simulink model "fourdrive_test"  (R2022b)
settings: Solver=FixedStepDiscrete  StartTime=0.0  StopTime=10.0  FixedStep=0.001  RelTol=1e-3  EnableMultiTasking=on
PreLoadFcn:
  | PowerOn_data
InitFcn:
  | EcoCoder_PreCheckLic();
undefined symbols (not defined in the file or in its folder): HV_Botton, Inverter_Button, SC_Closed
libraries: CoderSF_BSW_Libs x113, SF_CanService_Libs x24, CoderSF_ADC2Volt_Libs x10, simulink x2
(part 1 of 2)
settings Model: Param_HCUVersion=EV22297A  Creator=hxf  LastModifiedBy=34547
settings SolverCC: AlgebraicLoopSolver=TrustRegion  AutoInsertRateTranBlk=on
settings DataIOCC: SaveFormat=Structure  SignalLoggingSaveFormat=ModelDataLogs  SaveOutput=off  SignalLogging=off  DSMLogging=off  SaveTime=off  ReturnWorkspaceOutputs=off
settings OptimizationCC: DefaultParameterBehavior=Inlined  InlineInvariantSignals=on  EnhancedBackFolding=on  StrengthReduction=on  EnableMemcpy=off  PassReuseOutputArgsAs=Individual arguments  EfficientFloat2IntCast=on  LifeSpan=1  SimCompilerOptimization=on  OptimizeBlockOrder=speed  DifferentSizesBufferReuse=on  EfficientTunableParamExpr=on
settings DebuggingCC: AlgebraicLoopMsg=none  ArtificialAlgebraicLoopMsg=none  SaveWithDisabledLinksMsg=none  SaveWithParameterizedLinksMsg=none  CheckSSInitialOutputMsg=off  UnderspecifiedInitializationDetection=Classic  SignalResolutionControl=TryResolveAll  BlockPriorityViolationMsg=error  MinStepSizeMsg=none  InheritedTsInSrcMsg=none  MultiTaskDSMMsg=none  MultiTaskCondExecSysMsg=none  MultiTaskRateTransMsg=warning  TasksWithSamePriorityMsg=none  SigSpecEnsureSampleTimeMsg=none  IntegerOverflowMsg=error  Int32ToFloatConvMsg=none  ParameterPrecisionLossMsg=none  ParameterTunabilityLossMsg=none  FixptConstOverflowMsg=error  FcnCallInpInsideContextMsg=warning  UnconnectedInputMsg=error  UnconnectedOutputMsg=error  UnconnectedLineMsg=error  FrameProcessingCompatibilityMsg=none  BusObjectLabelMismatch=none  RootOutportRequireBusObject=none  UnknownTsInhSupMsg=none  ModelReferenceDataLoggingMessage=none  OperatingPointInterfaceChecksumMismatchMsg=none  SFUnusedDataAndEventsDiag=none  SFUnexpectedBacktrackingDiag=none  SFInvalidInputDataAccessInChartInitDiag=none  SFNoUnconditionalDefaultTransitionDiag=none  SFTransitionOutsideNaturalParentDiag=none  SFUnreachableExecutionPathDiag=none  SFMachineParentedDataDiag=warning  ArithmeticOperatorsInVariantConditions=warning
settings HardwareCC: ProdBitPerPointer=32  ProdBitPerSizeT=32  ProdBitPerPtrDiffT=32  ProdLargestAtomicFloat=None  ProdWordSize=32  ProdHWDeviceType=Infineon->TriCore
settings ModelReferenceCC: UpdateModelReferenceTargets=Force  EnableRefExpFcnMdlSchedulingChecks=on  ModelReferenceNumInstancesAllowed=Single  PropagateSignalLabelsOutOfModel=off
settings SFSimCC: SFSimEcho=off  MATLABDynamicMemAlloc=off  CustomCodeUndefinedFunction=UseInterfaceOnly
settings RTWCC: Description=Ecotrons TC27x  SystemTargetFile=EcoCoderTC27x.tlc  GenerateMakefile=off  TemplateMakefile=ert_default_tmf  RTWVerbose=off  RetainRTWFile=on  RTWCompilerOptimization=on
settings CodeAppCC: IgnoreCustomStorageClasses=off  OperatorAnnotations=on  CustomSymbolStrGlobalVar=$N$M  CustomSymbolStrType=$N$M  CustomSymbolStrFcn=$N$M  CustomSymbolStrFcnArg=$N$M  CustomSymbolStrBlkIO=$N$M  CustomSymbolStrMacro=$N$M
settings STFCustomTargetCC: UtilityFuncGeneration=Shared location  MultiwordLength=256  IncludeMdlTerminateFcn=off  CombineOutputUpdateFcns=on  SuppressErrorStatus=on  ERTCustomFileBanners=on  SupportComplex=off  SupportContinuousTime=off  SupportNonInlinedSFcns=off  MATLABClassNameForMDSCustomization=Simulink.SoftwareTarget.ERTCustomization  SystemTargetFile=EcoCoderTC27x.tlc
settings ERTTargetCC: UtilityFuncGeneration=Shared location  ParMdlRefBuildCompliant=off  CompOptLevelCompliant=off  ConcurrentExecutionCompliant=off  IncludeMdlTerminateFcn=off  SuppressErrorStatus=on  SupportComplex=off  RemoveResetFunc=off  ModelStepFunctionPrototypeControlCompliant=off  CPPClassGenCompliant=off  UseToolchainInfoCompliant=off  GenerateASAP2=on  InlinedParameterPlacement=NonHierarchical  ERTCustomFileTemplate=MPC5644A_file_process.tlc  ERTFilePackagingFormat=Compact  PreserveIfCondition=on  ConvertIfToSwitch=off  PreserveExternInFcnDecls=off  SuppressUnreachableDefaultCases=off

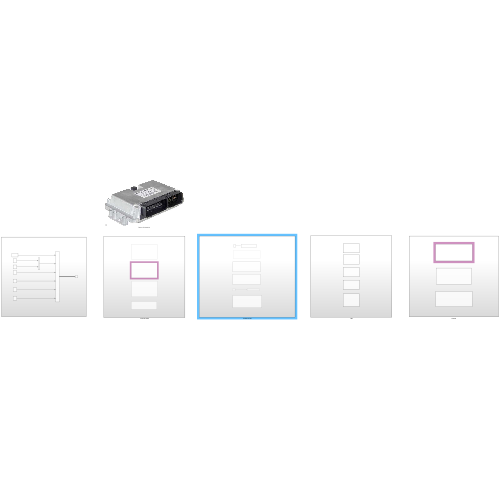
[thumbnail: Simulink's stored preview of the top-level diagram]
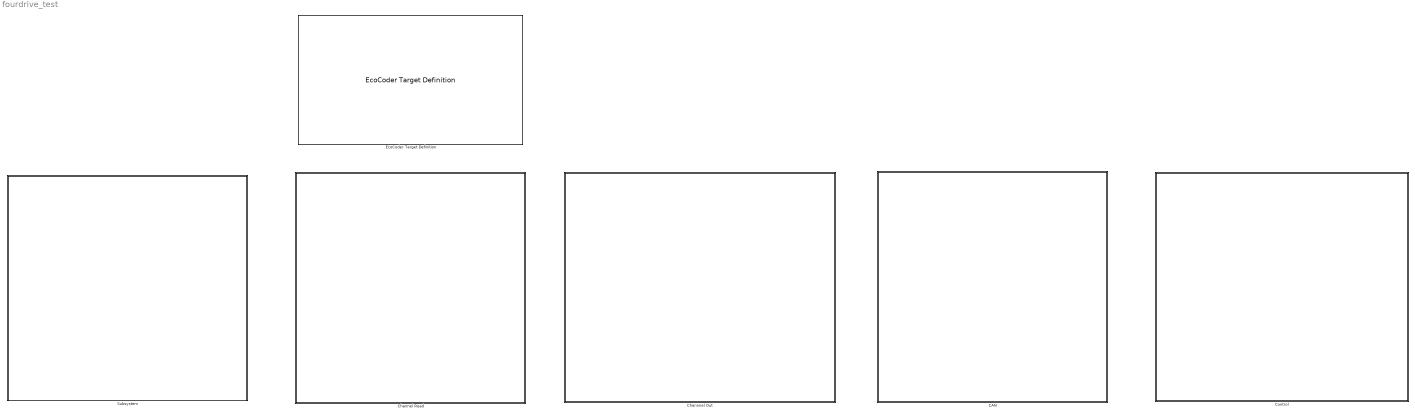
== system fourdrive_test ==
  CAN : Subsystem
  Channel Read : Subsystem
  Channnel Out : Subsystem
  Control : Subsystem
  EcoCoder Target Definition : CoderSF_BSW_Libs/EcoCoder Target Definition  targetECU=EV22297A  EcoCoderBlockID=T001_Target  enNoTriggerCall=on  flgBlockReduction=on  flgShowDebugDisp=off  flgDisTargetOutFIleCounter=off  flgClearAllOldFiles=on  tc275_cal_len=hex2dec('00008000')  ipVal='192.168.0.123'  userName='nvidia'  passWord='nvidia'  workSpace='~/cmake_ws'  libraryLink=''  enExt=on  portExt=17725  internal_flash=[hex2dec('00020000'),hex2dec('000E0000')]  cal_rom_phy=[hex2dec('00010000'),hex2dec('00002000')]  cal_ram_wp=[hex2dec('4000F000'),hex2dec('00002000')]  cal_ram_msm=[hex2dec('40000000'),hex2dec('00002000')]  var_ram_wp=[hex2dec('40002000'),hex2dec('0000D000')]  write_back_fixed_ram=[hex2dec('40011000'),hex2dec('00001000')]  write_back_unfixed_ram=[hex2dec('40012000'),hex2dec('00001000')]  stack=[hex2dec('40013000'),hex2dec('00001000')]
      settings: AttributesFormatString=Target :%<targetECU>
  Subsystem : Subsystem

== system fourdrive_test/CAN ==
  CAN Definition : Subsystem
  CAN Read : Subsystem
  CAN Write : Subsystem
  Fixed CCP Slave Definition : CoderSF_BSW_Libs/CCP/Fixed CCP Slave Definition  ccp_enSet=on  ccp_disASW=off  channel=CAN_B  stationaddressSet=hex2dec('0112')  croidSet=hex2dec('200')  dtoidSet=hex2dec('201')  daqidSet=[hex2dec('210') hex2dec('211') hex2dec('212') hex2dec('213')]  daqpidSet=[hex2dec('0') hex2dec('0') hex2dec('0') hex2dec('0')]  daqlenSet=[hex2dec('A') hex2dec('20') hex2dec('30') hex2dec('50')]  daqperSet=[10 20 100 200]  EcoCoderBlockID=C002_CCP21Conf
  Write CAN Measurement : Subsystem

== system fourdrive_test/Channel Read ==
  ADC : Subsystem
  DI : Subsystem

== system fourdrive_test/Channnel Out ==
  Constant1 : Constant  OutDataTypeStr=boolean
  DC板 : Subsystem
  Power Control Output : CoderSF_BSW_Libs/System Management Blocks/Power Control Output  channel=PWR5V3
  Terminator : Terminator
  水泵风扇 : Subsystem
  蜂鸣器 : Subsystem
  wires:
  Constant1/1 -> Power Control Output/1
  [Brake_angle_percent] -> Terminator/1

== system fourdrive_test/Control ==
  Motor_Enable : Subsystem
  StateMachine : Subsystem
  Torque_Control : Subsystem

== system fourdrive_test/Subsystem ==
  Bus Creator : BusCreator  Inputs=Wheelbase,Distribution of Axle Load,Front Length,Rear Length,Front Track Width,Rear Track Width
  Divide : Product  Inputs=*/
  Front Length : Constant  Value=0.79
  Front Mass : Constant  Value=110
  Front Track Width : Constant  Value=1.2
  Rear Length : Constant  Value=0.79
  Rear Mass : Constant  Value=135
  Rear Track Width : Constant  Value=1.16
  Terminator : Terminator
  Wheelbase : Constant  Value=1.58
  wires:
  Front Mass/1 -> Divide/1
  Rear Mass/1 -> Divide/2
  Divide/1 -> Bus Creator/2  "Distribution of Axle Load"
  Wheelbase/1 -> Bus Creator/1  "Wheelbase"
  Front Length/1 -> Bus Creator/3  "Front Length"
  Rear Length/1 -> Bus Creator/4  "Rear Length"
  Front Track Width/1 -> Bus Creator/5  "Front Track Width"
  Rear Track Width/1 -> Bus Creator/6  "Rear Track Width"
  Bus Creator/1 -> Terminator/1

== system fourdrive_test/CAN/CAN Definition ==
  CAN Channel Definition : CoderSF_BSW_Libs/CAN/CAN Channel Definition  channel=CAN_A  can_en=on  can_idfilter=off  can_rxextended=off  can_rxMask=hex2dec('7ff')  can_rxID=hex2dec('100')  can_baudrateIndex=250  can_txbuffer_size=200  can_rxbuffer_size=1  can_en_fd=off  nominalSamplePoint=7500  can_baudrateIndex_data=500  fastSamplePoint=7500  canfd_txbuffer_size=5  EcoCoderBlockID=C001_CANDef
  CAN Channel Definition1 : CoderSF_BSW_Libs/CAN/CAN Channel Definition  channel=CAN_B  can_en=on  can_idfilter=off  can_rxextended=off  can_rxMask=hex2dec('7ff')  can_rxID=hex2dec('100')  can_baudrateIndex=500  can_txbuffer_size=200  can_rxbuffer_size=1  can_en_fd=off  nominalSamplePoint=7500  can_baudrateIndex_data=500  fastSamplePoint=7500  canfd_txbuffer_size=5  EcoCoderBlockID=C001_CANDef
  CAN Channel Definition2 : CoderSF_BSW_Libs/CAN/CAN Channel Definition  channel=CAN_C  can_en=on  can_idfilter=off  can_rxextended=off  can_rxMask=hex2dec('7ff')  can_rxID=hex2dec('100')  can_baudrateIndex=500  can_txbuffer_size=20  can_rxbuffer_size=1  can_en_fd=off  nominalSamplePoint=7500  can_baudrateIndex_data=500  fastSamplePoint=7500  canfd_txbuffer_size=5  EcoCoderBlockID=C001_CANDef
  CAN Channel Definition3 : CoderSF_BSW_Libs/CAN/CAN Channel Definition  channel=CAN_D  can_en=on  can_idfilter=off  can_rxextended=off  can_rxMask=hex2dec('7ff')  can_rxID=hex2dec('100')  can_baudrateIndex=500  can_txbuffer_size=20  can_rxbuffer_size=1  can_en_fd=off  nominalSamplePoint=7500  can_baudrateIndex_data=500  fastSamplePoint=7500  canfd_txbuffer_size=5  EcoCoderBlockID=C001_CANDef
  CAN Channel Definition4 : CoderSF_BSW_Libs/CAN/CAN Channel Definition  channel=CAN_E  can_en=on  can_idfilter=off  can_rxextended=off  can_rxMask=hex2dec('7ff')  can_rxID=hex2dec('100')  can_baudrateIndex=250  can_txbuffer_size=20  can_rxbuffer_size=1  can_en_fd=off  nominalSamplePoint=7500  can_baudrateIndex_data=500  fastSamplePoint=7500  canfd_txbuffer_size=5  EcoCoderBlockID=C001_CANDef

== system fourdrive_test/CAN/CAN Read ==
  BMS_CAN : Subsystem
  Motor_CAN : Subsystem

== system fourdrive_test/CAN/CAN Write ==
  Send_To_Inverter : Subsystem
  Send_To_Recorder : Subsystem

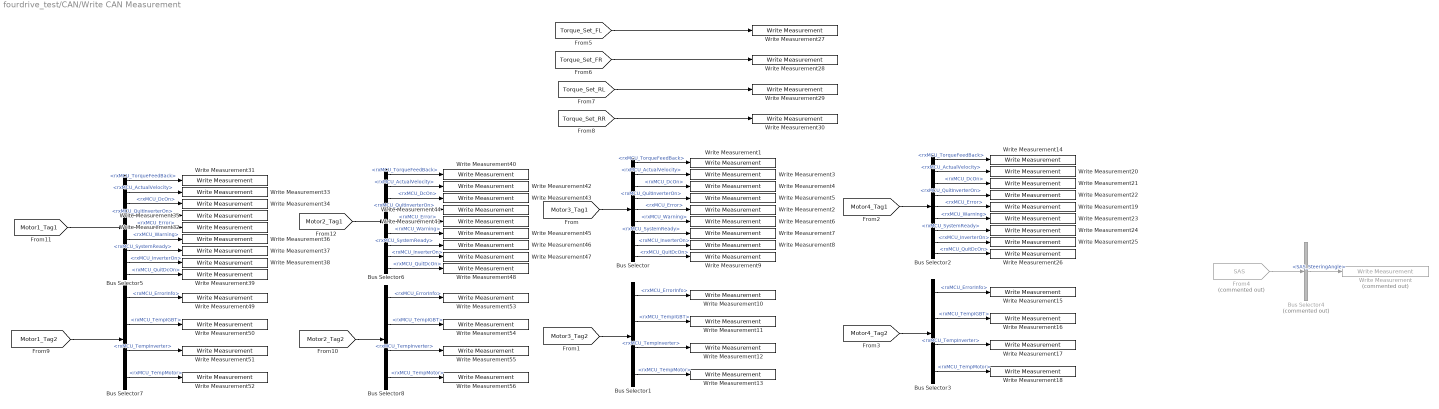
== system fourdrive_test/CAN/Write CAN Measurement ==
  Bus Selector{,2,5..6} (4 alike) : BusSelector  OutputSignals=rxMCU_TorqueFeedBack,rxMCU_ActualVelocity,rxMCU_DcOn,rxMCU_QuitInverterOn,rxMCU_Error,rxMCU_Warning,rxMCU_SystemReady,rxMCU_InverterOn,rxMCU_QuitDcOn
  Bus Selector{1,3,7..8} (4 alike) : BusSelector  OutputSignals=rxMCU_ErrorInfo,rxMCU_TempIGBT,rxMCU_TempInverter,rxMCU_TempMotor
  Bus Selector4 : BusSelector  Commented=on  OutputSignals=SAS_SteeringAngle
  From4 : From  Commented=on  GotoTag=SAS  TagVisibility=global
  Write Measurement : CoderSF_BSW_Libs/Calibration & Measurement/Write Measurement  Commented=on  variable_name=Steering_Angle  variable_value=0  variable_type=single  numD=1  unitStr=""  descStr=""
      settings: AttributesFormatString=type:%<variable_type> Dimensions:%<numD>
  Write Measurement1 : CoderSF_BSW_Libs/Calibration & Measurement/Write Measurement  variable_name=RL_Actual_Torque  variable_value=0  variable_type=single  numD=1  unitStr=""  descStr=""
      settings: AttributesFormatString=type:%<variable_type> Dimensions:%<numD>
  Write Measurement10 : CoderSF_BSW_Libs/Calibration & Measurement/Write Measurement  variable_name=RL_Error_Info  variable_value=0  variable_type=uint16  numD=1  unitStr=""  descStr=""
      settings: AttributesFormatString=type:%<variable_type> Dimensions:%<numD>
  Write Measurement11 : CoderSF_BSW_Libs/Calibration & Measurement/Write Measurement  variable_name=RL_TempIGBT  variable_value=0  variable_type=single  numD=1  unitStr=""  descStr=""
      settings: AttributesFormatString=type:%<variable_type> Dimensions:%<numD>
  Write Measurement12 : CoderSF_BSW_Libs/Calibration & Measurement/Write Measurement  variable_name=RL_TempInverter  variable_value=0  variable_type=single  numD=1  unitStr=""  descStr=""
      settings: AttributesFormatString=type:%<variable_type> Dimensions:%<numD>
  Write Measurement13 : CoderSF_BSW_Libs/Calibration & Measurement/Write Measurement  variable_name=RL_TempMotor  variable_value=0  variable_type=single  numD=1  unitStr=""  descStr=""
      settings: AttributesFormatString=type:%<variable_type> Dimensions:%<numD>
  Write Measurement14 : CoderSF_BSW_Libs/Calibration & Measurement/Write Measurement  variable_name=RR_Actual_Torque  variable_value=0  variable_type=single  numD=1  unitStr=""  descStr=""
      settings: AttributesFormatString=type:%<variable_type> Dimensions:%<numD>
  Write Measurement15 : CoderSF_BSW_Libs/Calibration & Measurement/Write Measurement  variable_name=RR_Error_Info  variable_value=0  variable_type=uint16  numD=1  unitStr=""  descStr=""
      settings: AttributesFormatString=type:%<variable_type> Dimensions:%<numD>
  Write Measurement16 : CoderSF_BSW_Libs/Calibration & Measurement/Write Measurement  variable_name=RR_TempIGBT  variable_value=0  variable_type=single  numD=1  unitStr=""  descStr=""
      settings: AttributesFormatString=type:%<variable_type> Dimensions:%<numD>
  Write Measurement17 : CoderSF_BSW_Libs/Calibration & Measurement/Write Measurement  variable_name=RR_TempInverter  variable_value=0  variable_type=single  numD=1  unitStr=""  descStr=""
      settings: AttributesFormatString=type:%<variable_type> Dimensions:%<numD>
  Write Measurement18 : CoderSF_BSW_Libs/Calibration & Measurement/Write Measurement  variable_name=RR_TempMotor  variable_value=0  variable_type=single  numD=1  unitStr=""  descStr=""
      settings: AttributesFormatString=type:%<variable_type> Dimensions:%<numD>
  Write Measurement19 : CoderSF_BSW_Libs/Calibration & Measurement/Write Measurement  variable_name=RR_Error  variable_value=0  variable_type=boolean  numD=1  unitStr=""  descStr=""
      settings: AttributesFormatString=type:%<variable_type> Dimensions:%<numD>
  Write Measurement2 : CoderSF_BSW_Libs/Calibration & Measurement/Write Measurement  variable_name=RL_Error  variable_value=0  variable_type=boolean  numD=1  unitStr=""  descStr=""
      settings: AttributesFormatString=type:%<variable_type> Dimensions:%<numD>
  Write Measurement20 : CoderSF_BSW_Libs/Calibration & Measurement/Write Measurement  variable_name=RR_Actual_Velocity  variable_value=0  variable_type=int16  numD=1  unitStr=""  descStr=""
      settings: AttributesFormatString=type:%<variable_type> Dimensions:%<numD>
  Write Measurement21 : CoderSF_BSW_Libs/Calibration & Measurement/Write Measurement  variable_name=RR_DCon  variable_value=0  variable_type=boolean  numD=1  unitStr=""  descStr=""
      settings: AttributesFormatString=type:%<variable_type> Dimensions:%<numD>
  Write Measurement22 : CoderSF_BSW_Libs/Calibration & Measurement/Write Measurement  variable_name=RR_Quit_Inverter_on  variable_value=0  variable_type=boolean  numD=1  unitStr=""  descStr=""
      settings: AttributesFormatString=type:%<variable_type> Dimensions:%<numD>
  Write Measurement23 : CoderSF_BSW_Libs/Calibration & Measurement/Write Measurement  variable_name=RR_Warning  variable_value=0  variable_type=boolean  numD=1  unitStr=""  descStr=""
      settings: AttributesFormatString=type:%<variable_type> Dimensions:%<numD>
  Write Measurement24 : CoderSF_BSW_Libs/Calibration & Measurement/Write Measurement  variable_name=RR_System_Ready  variable_value=0  variable_type=boolean  numD=1  unitStr=""  descStr=""
      settings: AttributesFormatString=type:%<variable_type> Dimensions:%<numD>
  Write Measurement25 : CoderSF_BSW_Libs/Calibration & Measurement/Write Measurement  variable_name=RR_Inverter_on  variable_value=0  variable_type=boolean  numD=1  unitStr=""  descStr=""
      settings: AttributesFormatString=type:%<variable_type> Dimensions:%<numD>
  Write Measurement26 : CoderSF_BSW_Libs/Calibration & Measurement/Write Measurement  variable_name=RR_QuitDCon  variable_value=0  variable_type=boolean  numD=1  unitStr=""  descStr=""
      settings: AttributesFormatString=type:%<variable_type> Dimensions:%<numD>
  Write Measurement27 : CoderSF_BSW_Libs/Calibration & Measurement/Write Measurement  variable_name=Torque_Set_FL  variable_value=0  variable_type=uint16  numD=1  unitStr=""  descStr=""
      settings: AttributesFormatString=type:%<variable_type> Dimensions:%<numD>
  Write Measurement28 : CoderSF_BSW_Libs/Calibration & Measurement/Write Measurement  variable_name=Torque_Set_FR  variable_value=0  variable_type=uint16  numD=1  unitStr=""  descStr=""
      settings: AttributesFormatString=type:%<variable_type> Dimensions:%<numD>
  Write Measurement29 : CoderSF_BSW_Libs/Calibration & Measurement/Write Measurement  variable_name=Torque_Set_RL  variable_value=0  variable_type=uint16  numD=1  unitStr=""  descStr=""
      settings: AttributesFormatString=type:%<variable_type> Dimensions:%<numD>
  Write Measurement3 : CoderSF_BSW_Libs/Calibration & Measurement/Write Measurement  variable_name=RL_Actual_Velocity  variable_value=0  variable_type=int16  numD=1  unitStr=""  descStr=""
      settings: AttributesFormatString=type:%<variable_type> Dimensions:%<numD>
  Write Measurement30 : CoderSF_BSW_Libs/Calibration & Measurement/Write Measurement  variable_name=Torque_Set_RR  variable_value=0  variable_type=uint16  numD=1  unitStr=""  descStr=""
      settings: AttributesFormatString=type:%<variable_type> Dimensions:%<numD>
  Write Measurement31 : CoderSF_BSW_Libs/Calibration & Measurement/Write Measurement  variable_name=FL_Actual_Torque  variable_value=0  variable_type=single  numD=1  unitStr=""  descStr=""
      settings: AttributesFormatString=type:%<variable_type> Dimensions:%<numD>
  Write Measurement32 : CoderSF_BSW_Libs/Calibration & Measurement/Write Measurement  variable_name=FL_Error  variable_value=0  variable_type=boolean  numD=1  unitStr=""  descStr=""
      settings: AttributesFormatString=type:%<variable_type> Dimensions:%<numD>
  Write Measurement33 : CoderSF_BSW_Libs/Calibration & Measurement/Write Measurement  variable_name=FL_Actual_Velocity  variable_value=0  variable_type=int16  numD=1  unitStr=""  descStr=""
      settings: AttributesFormatString=type:%<variable_type> Dimensions:%<numD>
  Write Measurement34 : CoderSF_BSW_Libs/Calibration & Measurement/Write Measurement  variable_name=FL_DCon  variable_value=0  variable_type=boolean  numD=1  unitStr=""  descStr=""
      settings: AttributesFormatString=type:%<variable_type> Dimensions:%<numD>
  Write Measurement35 : CoderSF_BSW_Libs/Calibration & Measurement/Write Measurement  variable_name=FL_Quit_Inverter_on  variable_value=0  variable_type=boolean  numD=1  unitStr=""  descStr=""
      settings: AttributesFormatString=type:%<variable_type> Dimensions:%<numD>
  Write Measurement36 : CoderSF_BSW_Libs/Calibration & Measurement/Write Measurement  variable_name=FL_Warning  variable_value=0  variable_type=boolean  numD=1  unitStr=""  descStr=""
      settings: AttributesFormatString=type:%<variable_type> Dimensions:%<numD>
  Write Measurement37 : CoderSF_BSW_Libs/Calibration & Measurement/Write Measurement  variable_name=FL_System_Ready  variable_value=0  variable_type=boolean  numD=1  unitStr=""  descStr=""
      settings: AttributesFormatString=type:%<variable_type> Dimensions:%<numD>
  Write Measurement38 : CoderSF_BSW_Libs/Calibration & Measurement/Write Measurement  variable_name=FL_Inverter_on  variable_value=0  variable_type=boolean  numD=1  unitStr=""  descStr=""
      settings: AttributesFormatString=type:%<variable_type> Dimensions:%<numD>
  Write Measurement39 : CoderSF_BSW_Libs/Calibration & Measurement/Write Measurement  variable_name=FL_QuitDCon  variable_value=0  variable_type=boolean  numD=1  unitStr=""  descStr=""
      settings: AttributesFormatString=type:%<variable_type> Dimensions:%<numD>
  Write Measurement4 : CoderSF_BSW_Libs/Calibration & Measurement/Write Measurement  variable_name=RL_DCon  variable_value=0  variable_type=boolean  numD=1  unitStr=""  descStr=""
      settings: AttributesFormatString=type:%<variable_type> Dimensions:%<numD>
  Write Measurement40 : CoderSF_BSW_Libs/Calibration & Measurement/Write Measurement  variable_name=FR_Actual_Torque  variable_value=0  variable_type=single  numD=1  unitStr=""  descStr=""
      settings: AttributesFormatString=type:%<variable_type> Dimensions:%<numD>
  Write Measurement41 : CoderSF_BSW_Libs/Calibration & Measurement/Write Measurement  variable_name=FR_Error  variable_value=0  variable_type=boolean  numD=1  unitStr=""  descStr=""
      settings: AttributesFormatString=type:%<variable_type> Dimensions:%<numD>
  Write Measurement42 : CoderSF_BSW_Libs/Calibration & Measurement/Write Measurement  variable_name=FR_Actual_Velocity  variable_value=0  variable_type=int16  numD=1  unitStr=""  descStr=""
      settings: AttributesFormatString=type:%<variable_type> Dimensions:%<numD>
  Write Measurement43 : CoderSF_BSW_Libs/Calibration & Measurement/Write Measurement  variable_name=FR_DCon  variable_value=0  variable_type=boolean  numD=1  unitStr=""  descStr=""
      settings: AttributesFormatString=type:%<variable_type> Dimensions:%<numD>
  Write Measurement44 : CoderSF_BSW_Libs/Calibration & Measurement/Write Measurement  variable_name=FR_Quit_Inverter_on  variable_value=0  variable_type=boolean  numD=1  unitStr=""  descStr=""
      settings: AttributesFormatString=type:%<variable_type> Dimensions:%<numD>
  Write Measurement45 : CoderSF_BSW_Libs/Calibration & Measurement/Write Measurement  variable_name=FR_Warning  variable_value=0  variable_type=boolean  numD=1  unitStr=""  descStr=""
      settings: AttributesFormatString=type:%<variable_type> Dimensions:%<numD>
  Write Measurement46 : CoderSF_BSW_Libs/Calibration & Measurement/Write Measurement  variable_name=FR_System_Ready  variable_value=0  variable_type=boolean  numD=1  unitStr=""  descStr=""
      settings: AttributesFormatString=type:%<variable_type> Dimensions:%<numD>
  Write Measurement47 : CoderSF_BSW_Libs/Calibration & Measurement/Write Measurement  variable_name=FR_Inverter_on  variable_value=0  variable_type=boolean  numD=1  unitStr=""  descStr=""
      settings: AttributesFormatString=type:%<variable_type> Dimensions:%<numD>
  Write Measurement48 : CoderSF_BSW_Libs/Calibration & Measurement/Write Measurement  variable_name=FR_QuitDCon  variable_value=0  variable_type=boolean  numD=1  unitStr=""  descStr=""
      settings: AttributesFormatString=type:%<variable_type> Dimensions:%<numD>
  Write Measurement49 : CoderSF_BSW_Libs/Calibration & Measurement/Write Measurement  variable_name=FL_Error_Info  variable_value=0  variable_type=uint16  numD=1  unitStr=""  descStr=""
      settings: AttributesFormatString=type:%<variable_type> Dimensions:%<numD>
  Write Measurement5 : CoderSF_BSW_Libs/Calibration & Measurement/Write Measurement  variable_name=RL_Quit_Inverter_on  variable_value=0  variable_type=boolean  numD=1  unitStr=""  descStr=""
      settings: AttributesFormatString=type:%<variable_type> Dimensions:%<numD>
  Write Measurement50 : CoderSF_BSW_Libs/Calibration & Measurement/Write Measurement  variable_name=FL_TempIGBT  variable_value=0  variable_type=single  numD=1  unitStr=""  descStr=""
      settings: AttributesFormatString=type:%<variable_type> Dimensions:%<numD>
  Write Measurement51 : CoderSF_BSW_Libs/Calibration & Measurement/Write Measurement  variable_name=FL_TempInverter  variable_value=0  variable_type=single  numD=1  unitStr=""  descStr=""
      settings: AttributesFormatString=type:%<variable_type> Dimensions:%<numD>
  Write Measurement52 : CoderSF_BSW_Libs/Calibration & Measurement/Write Measurement  variable_name=FL_TempMotor  variable_value=0  variable_type=single  numD=1  unitStr=""  descStr=""
      settings: AttributesFormatString=type:%<variable_type> Dimensions:%<numD>
  Write Measurement53 : CoderSF_BSW_Libs/Calibration & Measurement/Write Measurement  variable_name=FR_Error_Info  variable_value=0  variable_type=uint16  numD=1  unitStr=""  descStr=""
      settings: AttributesFormatString=type:%<variable_type> Dimensions:%<numD>
  Write Measurement54 : CoderSF_BSW_Libs/Calibration & Measurement/Write Measurement  variable_name=FR_TempIGBT  variable_value=0  variable_type=single  numD=1  unitStr=""  descStr=""
      settings: AttributesFormatString=type:%<variable_type> Dimensions:%<numD>
  Write Measurement55 : CoderSF_BSW_Libs/Calibration & Measurement/Write Measurement  variable_name=FR_TempInverter  variable_value=0  variable_type=single  numD=1  unitStr=""  descStr=""
      settings: AttributesFormatString=type:%<variable_type> Dimensions:%<numD>
  Write Measurement56 : CoderSF_BSW_Libs/Calibration & Measurement/Write Measurement  variable_name=FR_TempMotor  variable_value=0  variable_type=single  numD=1  unitStr=""  descStr=""
      settings: AttributesFormatString=type:%<variable_type> Dimensions:%<numD>
  Write Measurement6 : CoderSF_BSW_Libs/Calibration & Measurement/Write Measurement  variable_name=RL_Warning  variable_value=0  variable_type=boolean  numD=1  unitStr=""  descStr=""
      settings: AttributesFormatString=type:%<variable_type> Dimensions:%<numD>
  Write Measurement7 : CoderSF_BSW_Libs/Calibration & Measurement/Write Measurement  variable_name=RL_System_Ready  variable_value=0  variable_type=boolean  numD=1  unitStr=""  descStr=""
      settings: AttributesFormatString=type:%<variable_type> Dimensions:%<numD>
  Write Measurement8 : CoderSF_BSW_Libs/Calibration & Measurement/Write Measurement  variable_name=RL_Inverter_on  variable_value=0  variable_type=boolean  numD=1  unitStr=""  descStr=""
      settings: AttributesFormatString=type:%<variable_type> Dimensions:%<numD>
  Write Measurement9 : CoderSF_BSW_Libs/Calibration & Measurement/Write Measurement  variable_name=RL_QuitDCon  variable_value=0  variable_type=boolean  numD=1  unitStr=""  descStr=""
      settings: AttributesFormatString=type:%<variable_type> Dimensions:%<numD>
  wires:
  Bus Selector1/4 -> Write Measurement13/1  "<rxMCU_TempMotor>"
  Bus Selector/1 -> Write Measurement1/1  "<rxMCU_TorqueFeedBack>"
  Bus Selector2/9 -> Write Measurement26/1  "<rxMCU_QuitDcOn>"
  Bus Selector/2 -> Write Measurement3/1  "<rxMCU_ActualVelocity>"
  Bus Selector2/6 -> Write Measurement23/1  "<rxMCU_Warning>"
  Bus Selector/9 -> Write Measurement9/1  "<rxMCU_QuitDcOn>"
  Bus Selector/4 -> Write Measurement5/1  "<rxMCU_QuitInverterOn>"
  Bus Selector3/1 -> Write Measurement15/1  "<rxMCU_ErrorInfo>"
  Bus Selector3/3 -> Write Measurement17/1  "<rxMCU_TempInverter>"
  Bus Selector/3 -> Write Measurement4/1  "<rxMCU_DcOn>"
  [Motor3_Tag2] -> Bus Selector1/1
  Bus Selector/6 -> Write Measurement6/1  "<rxMCU_Warning>"
  Bus Selector/8 -> Write Measurement8/1  "<rxMCU_InverterOn>"
  Bus Selector/5 -> Write Measurement2/1  "<rxMCU_Error>"
  [Motor4_Tag2] -> Bus Selector3/1
  [Motor3_Tag1] -> Bus Selector/1
  Bus Selector2/2 -> Write Measurement20/1  "<rxMCU_ActualVelocity>"
  Bus Selector2/1 -> Write Measurement14/1  "<rxMCU_TorqueFeedBack>"
  Bus Selector3/4 -> Write Measurement18/1  "<rxMCU_TempMotor>"
  Bus Selector2/5 -> Write Measurement19/1  "<rxMCU_Error>"
  Bus Selector2/8 -> Write Measurement25/1  "<rxMCU_InverterOn>"
  Bus Selector3/2 -> Write Measurement16/1  "<rxMCU_TempIGBT>"
  Bus Selector1/3 -> Write Measurement12/1  "<rxMCU_TempInverter>"
  [Motor4_Tag1] -> Bus Selector2/1
  Bus Selector2/4 -> Write Measurement22/1  "<rxMCU_QuitInverterOn>"
  Bus Selector2/7 -> Write Measurement24/1  "<rxMCU_SystemReady>"
  Bus Selector2/3 -> Write Measurement21/1  "<rxMCU_DcOn>"
  Bus Selector1/2 -> Write Measurement11/1  "<rxMCU_TempIGBT>"
  Bus Selector1/1 -> Write Measurement10/1  "<rxMCU_ErrorInfo>"
  Bus Selector/7 -> Write Measurement7/1  "<rxMCU_SystemReady>"
  From4/1 -> Bus Selector4/1
  Bus Selector4/1 -> Write Measurement/1  "<SAS_SteeringAngle>"
  [Torque_Set_RR] -> Write Measurement30/1
  [Torque_Set_RL] -> Write Measurement29/1
  [Torque_Set_FR] -> Write Measurement28/1
  [Torque_Set_FL] -> Write Measurement27/1
  [Motor1_Tag1] -> Bus Selector5/1
  Bus Selector5/2 -> Write Measurement33/1  "<rxMCU_ActualVelocity>"
  Bus Selector5/5 -> Write Measurement32/1  "<rxMCU_Error>"
  Bus Selector5/3 -> Write Measurement34/1  "<rxMCU_DcOn>"
  Bus Selector5/1 -> Write Measurement31/1  "<rxMCU_TorqueFeedBack>"
  Bus Selector5/8 -> Write Measurement38/1  "<rxMCU_InverterOn>"
  Bus Selector5/4 -> Write Measurement35/1  "<rxMCU_QuitInverterOn>"
  Bus Selector5/6 -> Write Measurement36/1  "<rxMCU_Warning>"
  Bus Selector5/9 -> Write Measurement39/1  "<rxMCU_QuitDcOn>"
  Bus Selector5/7 -> Write Measurement37/1  "<rxMCU_SystemReady>"
  [Motor2_Tag1] -> Bus Selector6/1
  Bus Selector6/2 -> Write Measurement42/1  "<rxMCU_ActualVelocity>"
  Bus Selector6/5 -> Write Measurement41/1  "<rxMCU_Error>"
  Bus Selector6/3 -> Write Measurement43/1  "<rxMCU_DcOn>"
  Bus Selector6/1 -> Write Measurement40/1  "<rxMCU_TorqueFeedBack>"
  Bus Selector6/8 -> Write Measurement47/1  "<rxMCU_InverterOn>"
  Bus Selector6/4 -> Write Measurement44/1  "<rxMCU_QuitInverterOn>"
  Bus Selector6/6 -> Write Measurement45/1  "<rxMCU_Warning>"
  Bus Selector6/9 -> Write Measurement48/1  "<rxMCU_QuitDcOn>"
  Bus Selector6/7 -> Write Measurement46/1  "<rxMCU_SystemReady>"
  Bus Selector7/1 -> Write Measurement49/1  "<rxMCU_ErrorInfo>"
  Bus Selector7/2 -> Write Measurement50/1  "<rxMCU_TempIGBT>"
  Bus Selector7/3 -> Write Measurement51/1  "<rxMCU_TempInverter>"
  Bus Selector7/4 -> Write Measurement52/1  "<rxMCU_TempMotor>"
  [Motor1_Tag2] -> Bus Selector7/1
  Bus Selector8/1 -> Write Measurement53/1  "<rxMCU_ErrorInfo>"
  Bus Selector8/2 -> Write Measurement54/1  "<rxMCU_TempIGBT>"
  Bus Selector8/3 -> Write Measurement55/1  "<rxMCU_TempInverter>"
  Bus Selector8/4 -> Write Measurement56/1  "<rxMCU_TempMotor>"
  [Motor2_Tag2] -> Bus Selector8/1

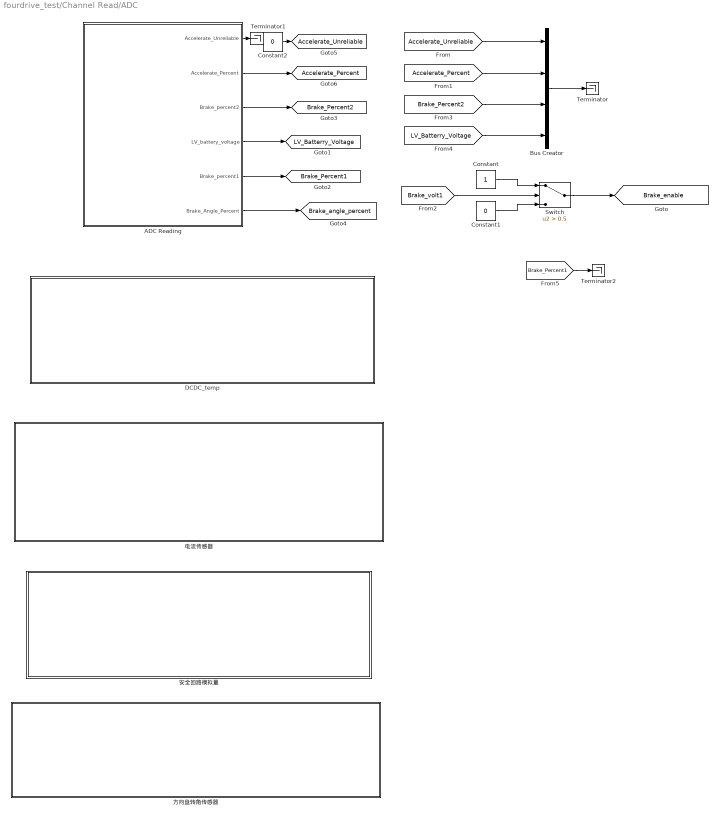
== system fourdrive_test/Channel Read/ADC ==
  "ADC Reading " : Subsystem
  Bus Creator : BusCreator  Inputs=4
  Constant : Constant
  Constant1 : Constant  Value=0
  Constant2 : Constant  Value=0
  DCDC_temp : Subsystem
  Switch : Switch  Criteria=u2 > Threshold  Threshold=0.5  SaturateOnIntegerOverflow=off  InputSameDT=off
  Terminator : Terminator
  Terminator1 : Terminator
  Terminator2 : Terminator
  安全回路模拟量 : Subsystem
  方向盘转角传感器 : Subsystem
  电流传感器 : Subsystem
  tag scope: Accelerate_Percent=global, Accelerate_Unreliable=global, Brake_Percent1=global, Brake_Percent2=global, Brake_angle_percent=global, Brake_enable=global, LV_Batterry_Voltage=global
  wires:
  [Brake_Percent2] -> Bus Creator/3
  [Accelerate_Percent] -> Bus Creator/2
  [Accelerate_Unreliable] -> Bus Creator/1
  "ADC Reading "/3(Brake_percent2) -> [Brake_Percent2]
  Bus Creator/1 -> Terminator/1
  "ADC Reading "/2(Accelerate_Percent) -> [Accelerate_Percent]
  [LV_Batterry_Voltage] -> Bus Creator/4
  "ADC Reading "/4(LV_battery_voltage) -> [LV_Batterry_Voltage]
  "ADC Reading "/5(Brake_percent1) -> [Brake_Percent1]
  [Brake_volt1] -> Switch/2
  Constant/1 -> Switch/1
  Constant1/1 -> Switch/3
  Switch/1 -> [Brake_enable]
  "ADC Reading "/6(Brake_Angle_Percent) -> [Brake_angle_percent]
  Constant2/1 -> [Accelerate_Unreliable]
  "ADC Reading "/1(Accelerate_Unreliable) -> Terminator1/1
  [Brake_Percent1] -> Terminator2/1

== system fourdrive_test/Channel Read/DI ==
  Bus Creator : BusCreator  Inputs=HV_Botton,Inverter_Button,SC_Closed
  Switch Input : CoderSF_BSW_Libs/Digital I//O/Switch Input  portNum=DI01
  Switch Input1 : CoderSF_BSW_Libs/Digital I//O/Switch Input  portNum=DI03
  Switch Input2 : CoderSF_BSW_Libs/Digital I//O/Switch Input  portNum=DI02
  Write Measurement : CoderSF_BSW_Libs/Calibration & Measurement/Write Measurement  variable_name=SC_Closed  variable_value=0  variable_type=boolean  numD=1  unitStr=""  descStr=""
      settings: AttributesFormatString=type:%<variable_type> Dimensions:%<numD>
  tag scope: DI=global
  wires:
  Bus Creator/1 -> [DI]
  Switch Input/1 -> Bus Creator/1  "HV_Botton"
  Switch Input1/1 -> Bus Creator/3, Write Measurement/1  "SC_Closed"
  Switch Input2/1 -> Bus Creator/2  "Inverter_Button"

== system fourdrive_test/Channnel Out/DC板 ==
  Chart : Stateflow chart  TreatAsAtomicUnit=on
  DC使能 : CoderSF_BSW_Libs/Digital I//O/Switch Output  channel=HSO06
  Write Measurement : CoderSF_BSW_Libs/Calibration & Measurement/Write Measurement  variable_name=DCDC_enable  variable_value=0  variable_type=boolean  numD=1  unitStr=""  descStr=""
      settings: AttributesFormatString=type:%<variable_type> Dimensions:%<numD>
  tag scope: DCDC_enable=global
  wires:
  Chart/1(DCDC_enable) -> [DCDC_enable]
  [DCDC_enable] -> Write Measurement/1, DC使能/1
  [Vehicle_Status] -> Chart/1(Vehicle_Status)
  [LV_Batterry_Voltage] -> Chart/2(LV_volt)

== system fourdrive_test/Channnel Out/水泵风扇 ==
  Compare To Constant : simulink/Logic and Bit Operations/Compare To Constant  relop===  const=1  OutDataTypeStr=boolean
  水泵使能 : CoderSF_BSW_Libs/Digital I//O/Switch Output  channel=HSO01
  wires:
  [Invertor_Enable] -> Compare To Constant/1
  Compare To Constant/1 -> 水泵使能/1

== system fourdrive_test/Channnel Out/蜂鸣器 ==
  AND1 : Logic  IconShape=distinctive  AllPortsSameDT=off  OutDataTypeStr=boolean
  Constant : Constant  Value=0  OutDataTypeStr=boolean
  Constant1 : Constant  OutDataTypeStr=boolean
  MATLAB Function : MATLAB Function  TreatAsAtomicUnit=on
  Switch : Switch  Criteria=u2 > Threshold  Threshold=100  OutDataTypeStr=boolean  SaturateOnIntegerOverflow=off  InputSameDT=off
  Write Measurement : CoderSF_BSW_Libs/Calibration & Measurement/Write Measurement  variable_name=buzzer  variable_value=0  variable_type=boolean  numD=1  unitStr=""  descStr=""
      settings: AttributesFormatString=type:%<variable_type> Dimensions:%<numD>
  蜂鸣器 : CoderSF_BSW_Libs/Digital I//O/Switch Output  channel=HSO08
  wires:
  Constant1/1 -> Switch/3
  Constant/1 -> Switch/1
  Switch/1 -> AND1/2
  MATLAB Function/1(count) -> Switch/2
  [Invertor_Enable] -> AND1/1, MATLAB Function/1(invertor)
  AND1/1 -> 蜂鸣器/1, Write Measurement/1

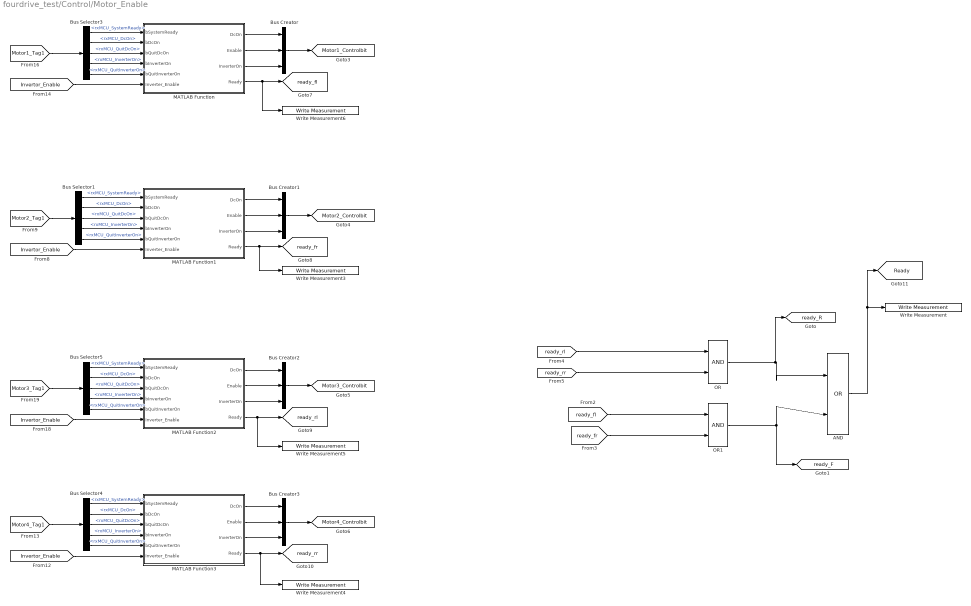
== system fourdrive_test/Control/Motor_Enable ==
  AND : Logic  Operator=OR  IconShape=distinctive  AllPortsSameDT=off  OutDataTypeStr=boolean
  Bus Creator{,1..3} (4 alike) : BusCreator  Inputs=3
  Bus Selector{1,3..5} (4 alike) : BusSelector  OutputSignals=rxMCU_SystemReady,rxMCU_DcOn,rxMCU_QuitDcOn,rxMCU_InverterOn,rxMCU_QuitInverterOn
  MATLAB Function : MATLAB Function  TreatAsAtomicUnit=on
  MATLAB Function1 : MATLAB Function  TreatAsAtomicUnit=on
  MATLAB Function2 : MATLAB Function  TreatAsAtomicUnit=on
  MATLAB Function3 : MATLAB Function  TreatAsAtomicUnit=on
  OR : Logic  IconShape=distinctive  AllPortsSameDT=off  OutDataTypeStr=boolean
  OR1 : Logic  IconShape=distinctive  AllPortsSameDT=off  OutDataTypeStr=boolean
  Write Measurement : CoderSF_BSW_Libs/Calibration & Measurement/Write Measurement  variable_name=Ready  variable_value=0  variable_type=boolean  numD=1  unitStr=""  descStr=""
      settings: AttributesFormatString=type:%<variable_type> Dimensions:%<numD>
  Write Measurement3 : CoderSF_BSW_Libs/Calibration & Measurement/Write Measurement  variable_name=ready_fr  variable_value=0  variable_type=int16  numD=1  unitStr=""  descStr=""
      settings: AttributesFormatString=type:%<variable_type> Dimensions:%<numD>
  Write Measurement4 : CoderSF_BSW_Libs/Calibration & Measurement/Write Measurement  variable_name=ready_rr  variable_value=0  variable_type=int16  numD=1  unitStr=""  descStr=""
      settings: AttributesFormatString=type:%<variable_type> Dimensions:%<numD>
  Write Measurement5 : CoderSF_BSW_Libs/Calibration & Measurement/Write Measurement  variable_name=ready_rl  variable_value=0  variable_type=int16  numD=1  unitStr=""  descStr=""
      settings: AttributesFormatString=type:%<variable_type> Dimensions:%<numD>
  Write Measurement6 : CoderSF_BSW_Libs/Calibration & Measurement/Write Measurement  variable_name=ready_fl  variable_value=0  variable_type=int16  numD=1  unitStr=""  descStr=""
      settings: AttributesFormatString=type:%<variable_type> Dimensions:%<numD>
  tag scope: Motor1_Controlbit=global, Motor2_Controlbit=global, Motor3_Controlbit=global, Motor4_Controlbit=global, Ready=global, ready_F=global, ready_R=global, ready_fl=global, ready_fr=global, ready_rl=global, ready_rr=global
  wires:
  MATLAB Function/2(Enable) -> Bus Creator/2
  [Invertor_Enable] -> MATLAB Function/6(Inverter_Enable)
  Bus Selector1/4 -> MATLAB Function1/4(bInverterOn)  "<rxMCU_InverterOn>"
  [Invertor_Enable] -> MATLAB Function2/6(Inverter_Enable)
  Bus Selector3/5 -> MATLAB Function/5(bQuitInverterOn)  "<rxMCU_QuitInverterOn>"
  Bus Selector4/4 -> MATLAB Function3/4(bInverterOn)  "<rxMCU_InverterOn>"
  MATLAB Function/3(InverterOn) -> Bus Creator/3
  MATLAB Function3/4(Ready) -> Write Measurement4/1, [ready_rr]
  AND/1 -> [Ready], Write Measurement/1
  MATLAB Function/4(Ready) -> Write Measurement6/1, [ready_fl]
  Bus Selector3/2 -> MATLAB Function/2(bDcOn)  "<rxMCU_DcOn>"
  Bus Creator3/1 -> [Motor4_Controlbit]
  Bus Selector1/3 -> MATLAB Function1/3(bQuitDcOn)  "<rxMCU_QuitDcOn>"
  Bus Selector4/2 -> MATLAB Function3/2(bDcOn)  "<rxMCU_DcOn>"
  Bus Creator/1 -> [Motor1_Controlbit]
  Bus Selector4/1 -> MATLAB Function3/1(bSystemReady)  "<rxMCU_SystemReady>"
  Bus Selector1/2 -> MATLAB Function1/2(bDcOn)  "<rxMCU_DcOn>"
  MATLAB Function1/4(Ready) -> Write Measurement3/1, [ready_fr]
  [Invertor_Enable] -> MATLAB Function3/6(Inverter_Enable)
  Bus Selector5/3 -> MATLAB Function2/3(bQuitDcOn)  "<rxMCU_QuitDcOn>"
  MATLAB Function1/1(DcOn) -> Bus Creator1/1
  Bus Selector5/5 -> MATLAB Function2/5(bQuitInverterOn)  "<rxMCU_QuitInverterOn>"
  MATLAB Function3/3(InverterOn) -> Bus Creator3/3
  Bus Selector3/3 -> MATLAB Function/3(bQuitDcOn)  "<rxMCU_QuitDcOn>"
  MATLAB Function2/4(Ready) -> Write Measurement5/1, [ready_rl]
  MATLAB Function2/2(Enable) -> Bus Creator2/2
  MATLAB Function1/2(Enable) -> Bus Creator1/2
  [Motor4_Tag1] -> Bus Selector4/1
  Bus Selector3/4 -> MATLAB Function/4(bInverterOn)  "<rxMCU_InverterOn>"
  MATLAB Function/1(DcOn) -> Bus Creator/1
  Bus Selector5/2 -> MATLAB Function2/2(bDcOn)  "<rxMCU_DcOn>"
  Bus Selector3/1 -> MATLAB Function/1(bSystemReady)  "<rxMCU_SystemReady>"
  MATLAB Function1/3(InverterOn) -> Bus Creator1/3
  [Motor1_Tag1] -> Bus Selector3/1
  MATLAB Function2/1(DcOn) -> Bus Creator2/1
  [Invertor_Enable] -> MATLAB Function1/6(Inverter_Enable)
  MATLAB Function3/2(Enable) -> Bus Creator3/2
  Bus Selector5/4 -> MATLAB Function2/4(bInverterOn)  "<rxMCU_InverterOn>"
  MATLAB Function2/3(InverterOn) -> Bus Creator2/3
  Bus Selector4/5 -> MATLAB Function3/5(bQuitInverterOn)  "<rxMCU_QuitInverterOn>"
  [Motor3_Tag1] -> Bus Selector5/1
  Bus Selector5/1 -> MATLAB Function2/1(bSystemReady)  "<rxMCU_SystemReady>"
  Bus Selector1/1 -> MATLAB Function1/1(bSystemReady)  "<rxMCU_SystemReady>"
  Bus Selector1/5 -> MATLAB Function1/5(bQuitInverterOn)  "<rxMCU_QuitInverterOn>"
  [Motor2_Tag1] -> Bus Selector1/1
  Bus Creator2/1 -> [Motor3_Controlbit]
  Bus Creator1/1 -> [Motor2_Controlbit]
  Bus Selector4/3 -> MATLAB Function3/3(bQuitDcOn)  "<rxMCU_QuitDcOn>"
  MATLAB Function3/1(DcOn) -> Bus Creator3/1
  [ready_rl] -> OR/1
  [ready_fl] -> OR1/1
  [ready_fr] -> OR1/2
  [ready_rr] -> OR/2
  OR/1 -> [ready_R], AND/1
  OR1/1 -> [ready_F], AND/2

== system fourdrive_test/Control/StateMachine ==
  Bus Selector2 : BusSelector  OutputSignals=HV_Botton,Inverter_Button,SC_Closed
  Chart : Stateflow chart  TreatAsAtomicUnit=on
  NOT : Logic  Operator=NOT  IconShape=distinctive  AllPortsSameDT=off  OutDataTypeStr=boolean
  NOT1 : Logic  Operator=NOT  IconShape=distinctive  AllPortsSameDT=off  OutDataTypeStr=boolean
  Switch Output1 : CoderSF_BSW_Libs/Digital I//O/Switch Output  channel=HSO09
  Write Measurement : CoderSF_BSW_Libs/Calibration & Measurement/Write Measurement  variable_name=Vehicle_Status  variable_value=0  variable_type=single  numD=1  unitStr=""  descStr=""
      settings: AttributesFormatString=type:%<variable_type> Dimensions:%<numD>
  Write Measurement1 : CoderSF_BSW_Libs/Calibration & Measurement/Write Measurement  variable_name=HV_Enable  variable_value=0  variable_type=boolean  numD=1  unitStr=""  descStr=""
      settings: AttributesFormatString=type:%<variable_type> Dimensions:%<numD>
  Write Measurement2 : CoderSF_BSW_Libs/Calibration & Measurement/Write Measurement  variable_name=Invertor_Enable  variable_value=0  variable_type=boolean  numD=1  unitStr=""  descStr=""
      settings: AttributesFormatString=type:%<variable_type> Dimensions:%<numD>
  tag scope: HV_Enable=global, Invertor_Enable=global, Vehicle_Status=global
  wires:
  Bus Selector2/3 -> Chart/3(SC_Closed)  "<SC_Closed>"
  Chart/2(HV_Enable) -> [HV_Enable]
  Bus Selector2/1 -> NOT/1  "<HV_Botton>"
  Chart/1(Vehicle_Status) -> [Vehicle_Status]
  Chart/3(Invertor_Enable) -> [Invertor_Enable]
  [DI] -> Bus Selector2/1
  [Vehicle_Status] -> Write Measurement/1
  [Accelerate_Unreliable] -> Chart/4(Pedal_Unrelible)
  [Invertor_Enable] -> Write Measurement2/1
  [HV_Enable] -> Switch Output1/1, Write Measurement1/1
  NOT/1 -> Chart/1(HV_Button)
  Bus Selector2/2 -> NOT1/1  "<Inverter_Button>"
  NOT1/1 -> Chart/2(Invertor_Button)
  [Brake_enable] -> Chart/5(Brake_enable)
  [Accelerate_Percent] -> Chart/6(Accelerate_Percent)

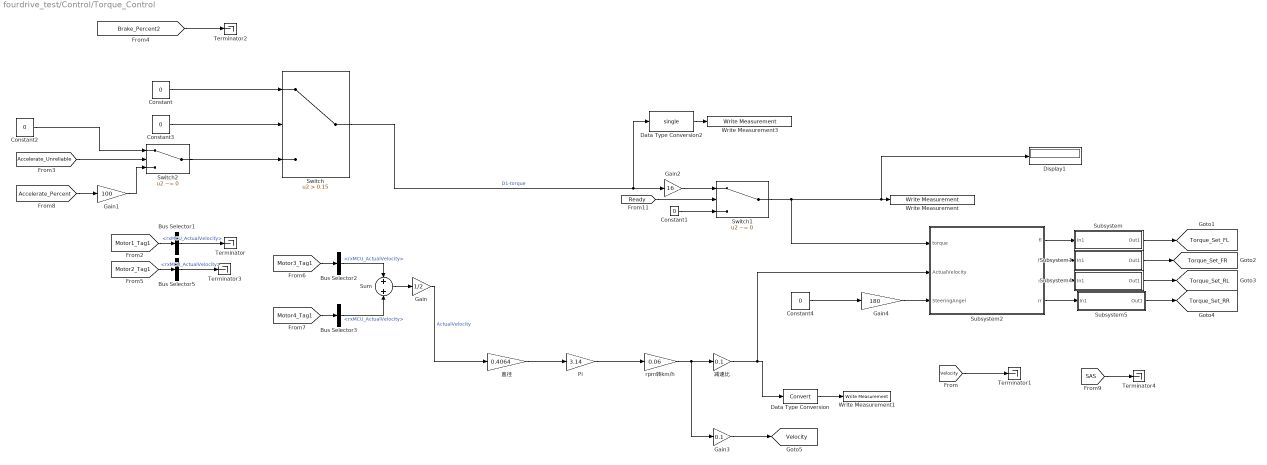
== system fourdrive_test/Control/Torque_Control ==
  Bus Selector{1..3,5} (4 alike) : BusSelector  OutputSignals=rxMCU_ActualVelocity
  Constant{,1..3} (4 alike) : Constant  Value=0
  Constant4 : Constant  Value=0  OutDataTypeStr=single
  Data Type Conversion : DataTypeConversion  SaturateOnIntegerOverflow=off  RndMeth=Floor
  Data Type Conversion2 : DataTypeConversion  OutDataTypeStr=single  SaturateOnIntegerOverflow=off  RndMeth=Floor
  Display1 : Display
  Gain : Gain  Gain=1/2  ParamDataTypeStr=uint16  OutDataTypeStr=uint16
  Gain1 : Gain  Gain=100
  Gain2 : Gain  Gain=16
  Gain3 : Gain  Gain=0.1  ParamDataTypeStr=uint16
  Gain4 : Gain  Gain=180
  Pi : Gain  Gain=3.14  OutDataTypeStr=single
  Subsystem : Subsystem
  Subsystem1 : Subsystem
  Subsystem2 : Subsystem
  Subsystem4 : Subsystem
  Subsystem5 : Subsystem
  Sum : Sum
  Switch : Switch  Criteria=u2 > Threshold  Threshold=0.15  SaturateOnIntegerOverflow=off  InputSameDT=off
  Switch1 : Switch  Criteria=u2 ~= 0  Threshold=0.1  OutDataTypeStr=int16  SaturateOnIntegerOverflow=off  InputSameDT=off
  Switch2 : Switch  Criteria=u2 ~= 0  SaturateOnIntegerOverflow=off  InputSameDT=off
  Terminator{,1..4} (5 alike) : Terminator
  Write Measurement : CoderSF_BSW_Libs/Calibration & Measurement/Write Measurement  variable_name=torque_output  variable_value=0  variable_type=int16  numD=1  unitStr=""  descStr=""
      settings: AttributesFormatString=type:%<variable_type> Dimensions:%<numD>
  Write Measurement1 : CoderSF_BSW_Libs/Calibration & Measurement/Write Measurement  variable_name=actual_velocity  variable_value=0  variable_type=single  numD=1  unitStr=""  descStr=""
      settings: AttributesFormatString=type:%<variable_type> Dimensions:%<numD>
  Write Measurement3 : CoderSF_BSW_Libs/Calibration & Measurement/Write Measurement  variable_name=percent_out  variable_value=0  variable_type=single  numD=1  unitStr=""  descStr=""
      settings: AttributesFormatString=type:%<variable_type> Dimensions:%<numD>
  rpm转km/h : Gain  Gain=0.06  OutDataTypeStr=single
  减速比 : Gain  Gain=0.1  OutDataTypeStr=single
  直径 : Gain  Gain=0.4064  OutDataTypeStr=single
  tag scope: Torque_Set_FL=global, Torque_Set_FR=global, Torque_Set_RL=global, Torque_Set_RR=global, Velocity=global
  wires:
  Constant1/1 -> Switch1/3
  Switch/1 -> Data Type Conversion2/1, Gain2/1  "D1-torque"
  Gain2/1 -> Switch1/1
  Sum/1 -> Gain/1
  [Motor3_Tag1] -> Bus Selector2/1
  [Motor4_Tag1] -> Bus Selector3/1
  Gain/1 -> 直径/1  "ActualVelocity"
  Constant/1 -> Switch/1
  Gain1/1 -> Switch2/3
  [Accelerate_Percent] -> Gain1/1
  [Accelerate_Unreliable] -> Switch2/2
  Constant2/1 -> Switch2/1
  Switch2/1 -> Switch/3
  直径/1 -> Pi/1
  Pi/1 -> rpm转km/h/1
  rpm转km/h/1 -> Gain3/1, 减速比/1
  Bus Selector2/1 -> Sum/1  "<rxMCU_ActualVelocity>"
  Data Type Conversion/1 -> Write Measurement1/1
  减速比/1 -> Data Type Conversion/1, Subsystem2/2(ActualVelocity)
  Data Type Conversion2/1 -> Write Measurement3/1
  Bus Selector5/1 -> Terminator3/1  "<rxMCU_ActualVelocity>"
  [Motor2_Tag1] -> Bus Selector5/1
  [Motor1_Tag1] -> Bus Selector1/1
  Bus Selector1/1 -> Terminator/1  "<rxMCU_ActualVelocity>"
  Bus Selector3/1 -> Sum/2  "<rxMCU_ActualVelocity>"
  Switch1/1 -> Subsystem2/1(torque), Display1/1, Write Measurement/1
  [Ready] -> Switch1/2
  [Velocity] -> Terminator1/1
  Constant3/1 -> Switch/2
  [Brake_Percent2] -> Terminator2/1
  Constant4/1 -> Gain4/1
  Subsystem2/3(rl) -> Subsystem4/1(In1)
  Subsystem2/4(rr) -> Subsystem5/1(In1)
  Subsystem2/2(fr) -> Subsystem1/1(In1)
  Subsystem2/1(fl) -> Subsystem/1(In1)
  Gain3/1 -> [Velocity]
  Gain4/1 -> Subsystem2/3(SteeringAngel)
  Subsystem/1(Out1) -> [Torque_Set_FL]
  Subsystem1/1(Out1) -> [Torque_Set_FR]
  Subsystem4/1(Out1) -> [Torque_Set_RL]
  Subsystem5/1(Out1) -> [Torque_Set_RR]
  [SAS] -> Terminator4/1

== system fourdrive_test/CAN/CAN Read/BMS_CAN ==
  Bus Creator : BusCreator  Inputs=9
  Bus Creator1 : BusCreator  Inputs=7
  Bus Creator2 : BusCreator  Inputs=9
  Read CAN Message : SF_CanService_Libs/Read CAN Message  typeCAN=Connected  channel=CAN_E  mEn=off  msgInfo=BCU_HCU_INFO_v3  msgItermStore=BMS_HCU_INFO  msgIterm=BMS_HCU_INFO  valid=on  stale=on  motoBit=off  setSignalName=on  flgCustomMonitorVariableRules=on  defineSignalName=off  prefixSignal=''  flgValTest=off  flgNoFixed=on  tSample=Task_Inherit  modeCode=Parameterless
  Read CAN Message1 : SF_CanService_Libs/Read CAN Message  typeCAN=Connected  channel=CAN_E  mEn=off  msgInfo=BCU_HCU_INFO_v3  msgItermStore=BMS_HCU_MAXV  msgIterm=BMS_HCU_MAXV  valid=on  stale=on  motoBit=off  setSignalName=on  flgCustomMonitorVariableRules=on  defineSignalName=off  prefixSignal=''  flgValTest=off  flgNoFixed=on  tSample=Task_Inherit  modeCode=Parameterless
  Read CAN Message2 : SF_CanService_Libs/Read CAN Message  typeCAN=Connected  channel=CAN_E  mEn=off  msgInfo=BCU_HCU_INFO_v3  msgItermStore=BMS_HCU_MAXT  msgIterm=BMS_HCU_MAXT  valid=on  stale=on  motoBit=off  setSignalName=on  flgCustomMonitorVariableRules=on  defineSignalName=off  prefixSignal=''  flgValTest=off  flgNoFixed=on  tSample=Task_Inherit  modeCode=Parameterless
  Terminator : Terminator
  Terminator1 : Terminator
  Terminator2 : Terminator
  tag scope: BMS_INFO=global, BMS_MAXT=global, BMS_MAXV=global
  wires:
  Bus Creator/1 -> [BMS_INFO]
  Read CAN Message/3 -> Bus Creator/3  "BatVoltage"
  Read CAN Message/6 -> Bus Creator/6  "BatSoc"
  Read CAN Message/1 -> Bus Creator/1
  Read CAN Message/5 -> Bus Creator/5  "BatSoh"
  Read CAN Message/2 -> Bus Creator/2
  Read CAN Message/4 -> Bus Creator/4  "BatState"
  Read CAN Message/9 -> Bus Creator/9  "BatAlmLv"
  Read CAN Message/7 -> Bus Creator/7  "BatLife"
  Read CAN Message/8 -> Bus Creator/8  "BatCurrent"
  Read CAN Message1/1 -> Bus Creator1/1
  Read CAN Message1/2 -> Bus Creator1/2
  Read CAN Message1/3 -> Bus Creator1/3  "Unused_2"
  Read CAN Message1/4 -> Bus Creator1/4  "MinCellVoltNo"
  Read CAN Message1/5 -> Bus Creator1/5  "MaxCellVoltNo"
  Read CAN Message1/6 -> Bus Creator1/6  "MinCellVolt"
  Bus Creator1/1 -> [BMS_MAXV]
  Read CAN Message2/6 -> Bus Creator2/6  "MinTempNo"
  Read CAN Message2/1 -> Bus Creator2/1
  Read CAN Message2/4 -> Bus Creator2/4  "Heating_Ctl"
  Read CAN Message2/5 -> Bus Creator2/5  "Cooling_Ctl"
  Read CAN Message2/3 -> Bus Creator2/3  "Unused_1"
  Read CAN Message2/2 -> Bus Creator2/2
  Bus Creator2/1 -> [BMS_MAXT]
  Read CAN Message1/7 -> Bus Creator1/7  "MaxCellVolt"
  Read CAN Message2/7 -> Bus Creator2/7  "MaxTempNo"
  Read CAN Message2/8 -> Bus Creator2/8  "MinTemp"
  Read CAN Message2/9 -> Bus Creator2/9  "MaxTemp"
  [BMS_MAXV] -> Terminator/1
  [BMS_MAXT] -> Terminator1/1
  [BMS_INFO] -> Terminator2/1
